simulink model "nonlinearModel"  (R2022b)
settings: Solver=VariableStepAuto  StartTime=0.0  StopTime=100  RelTol=1e-3
values from neighbouring files (symbols this model uses):
  C = zeros(3,6)    [sim1_PartD.m]    (also in sim2_PartF.m = [1,0,0,0,0,0; sim3_partG_part1.m = CC(var_sel,:); sim4_partG_part2.m = CC(var_sel,:))
  D = zeros(3,1)    [sim1_PartD.m]    (also in sim2_PartF.m = zeros(size(C,1),1); sim3_partG_part1.m = zeros(n_output_var,1); sim4_partG_part2.m = zeros(n_output_var,1))
  init_state = [x0,xd0,theta1_0,theta1_d0,theta2_0,theta2_d0]'    [sim1_PartD.m]    (also in sim2_PartF.m = [5,-0.5,20/180*pi,-0.5,-20/180*pi,0.5]'; sim3_partG_part1.m = [5,-0.5,20/180*pi,-0.5,-20/180*pi,0.5]'; sim4_partG_part2.m = [0,0,0,0,0,0]')
  K = -K    [sim1_PartD.m]    (also in sim3_partG_part1.m)
settings Model: Creator=liuji  LastModifiedBy=liuji

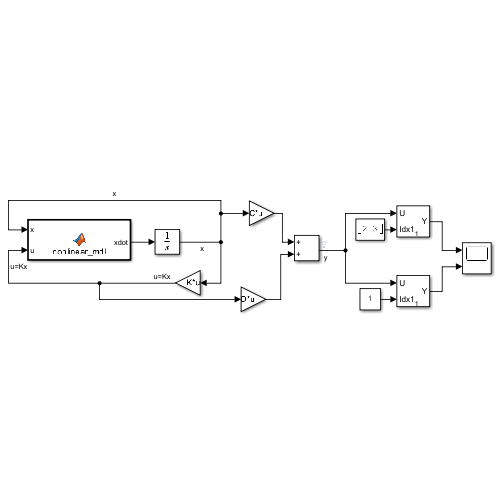
[thumbnail: Simulink's stored preview of the top-level diagram]
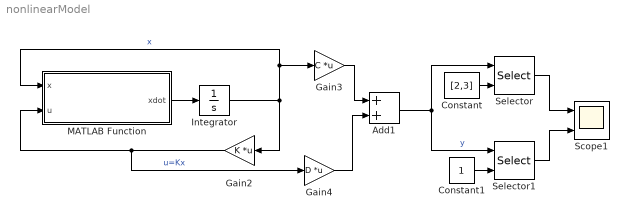
== system nonlinearModel ==
  Add1 : Sum
  Constant : Constant  Value=[2,3]
  Constant1 : Constant
  Gain2 : Gain  Gain=K  Multiplication=Matrix(K*u)
  Gain3 : Gain  Gain=C  Multiplication=Matrix(K*u)
  Gain4 : Gain  Gain=D  Multiplication=Matrix(K*u)
  Integrator : Integrator  InitialCondition=init_state
  MATLAB Function : MATLAB Function  TreatAsAtomicUnit=on
  Scope1 : Scope  NumInputPorts=2
  Selector : Selector  InputPortWidth=3  IndexOptions=Index vector (port)  Indices=[1 3]  OutputSizes=1
  Selector1 : Selector  InputPortWidth=3  IndexOptions=Index vector (port)  Indices=[1 3]  OutputSizes=1
  wires:
  Integrator/1 -> MATLAB Function/1(x), Gain3/1, Gain2/1  "x"
  Gain2/1 -> Gain4/1, MATLAB Function/2(u)  "u=Kx"
  Gain3/1 -> Add1/1
  Gain4/1 -> Add1/2
  Add1/1 -> Selector/1, Selector1/1  "y"
  Constant/1 -> Selector/2
  Selector/1 -> Scope1/1
  Constant1/1 -> Selector1/2
  Selector1/1 -> Scope1/2
  MATLAB Function/1(xdot) -> Integrator/1

== matlab function nonlinearModel/MATLAB Function ==
  data: x input; u input; xdot output; param parameter
function xdot = nonlinear_mdl(x,u,param)
    % implements the original dyanmics model
    M = param.M;
    m1 = param.m1;
    m2 = param.m2;
    l1 = param.l1;
    l2 = param.l2;
    g = param.g;
    x1 = x(1);
    x2 = x(2);
    x3 = x(3);
    x4 = x(4);
    x5 = x(5);
    x6 = x(6);
    xdot = zeros(6,1);
    xdot(1) = x2;
    xdot(2) = 1/(M + m1*sin(x3)^2 + m2*sin(x5)^2)*...
        (m1*g*sin(x3)*cos(x3) + m1*l1*x4^2*sin(x3) + m2*g*sin(x5)*cos(x5) + m2*l2*x6^2*sin(x5) + u);
    xdot(3) = x4;
    xdot(4) = -1/(l1*( M + m1*sin(x3)^2 + m2*sin(x5)^2 ))*...
        (m1*g*sin(x3) + m2*g*sin(x5)*cos(x3-x5) + m1*l1*x4^2*sin(x3)*cos(x3) + m2*l2*x6^2*sin(x5)*cos(x3) + ...
        M*g*sin(x3) + u*cos(x3));
    xdot(5) = x6;
    xdot(6) = -1/(l2*( M + m1*sin(x3)^2 + m2*sin(x5)^2 ))*...
        (m2*g*sin(x5) + m1*g*sin(x3)*cos(x3-x5) + m1*l1*x4^2*sin(x3)*cos(x5) + m2*l2*x6^2*sin(x5)*cos(x5) + ...
        M*g*sin(x5) + u*cos(x5));
